simulink model "estimacion1"  (R2024a)
settings: Solver=VariableStepAuto  StartTime=0.0  StopTime=100  RelTol=1e-3
libraries: simulink x1
settings Model: Creator=nicolas  LastModifiedBy=nicolas

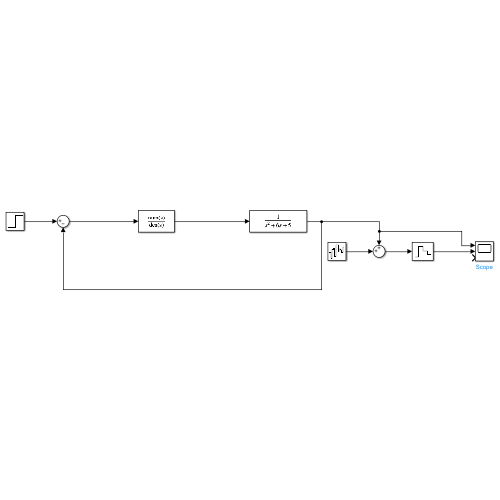
[thumbnail: Simulink's stored preview of the top-level diagram]
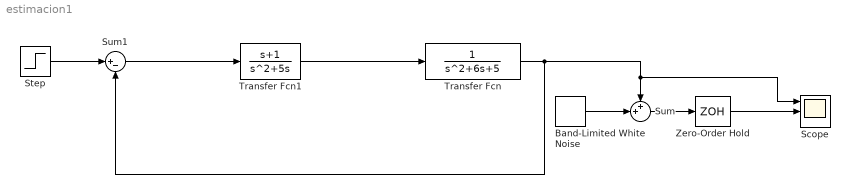
== system estimacion1 ==
  Band-Limited White Noise : simulink/Sources/Band-Limited White Noise  Cov=[0.0001]  Ts=0.2  seed=[23341]
  Scope : Scope  NumInputPorts=3
  Step : Step  SampleTime=0
  Sum : Sum  Inputs=++|
  Sum1 : Sum  Inputs=|+-
  Transfer Fcn : TransferFcn  Denominator=[1 6 5]
  Transfer Fcn1 : TransferFcn  Numerator=[1 1]  Denominator=[1 5 0]
  Zero-Order Hold : ZeroOrderHold  SampleTime=-1
  wires:
  Transfer Fcn/1 -> Sum/1, Scope/1, Sum1/2
  Band-Limited White Noise/1 -> Sum/2
  Transfer Fcn1/1 -> Transfer Fcn/1
  Sum1/1 -> Transfer Fcn1/1
  Step/1 -> Sum1/1
  Sum/1 -> Zero-Order Hold/1
  Zero-Order Hold/1 -> Scope/2
